simulink model "gm_CORDIC"  (R2016b)
settings: Solver=VariableStepAuto  StartTime=0.0  StopTime=20  RelTol=1e-3
undefined symbols (not defined in the file or in its folder): pht, scale, x_in, y_in, z_in
libraries: hdlsllib x24
settings Model: Creator=Arthur  LastModifiedBy=Arthur
settings OptimizationCC: BlockReduction=off  ConditionallyExecuteInputs=off
settings DebuggingCC: InheritedTsInSrcMsg=none

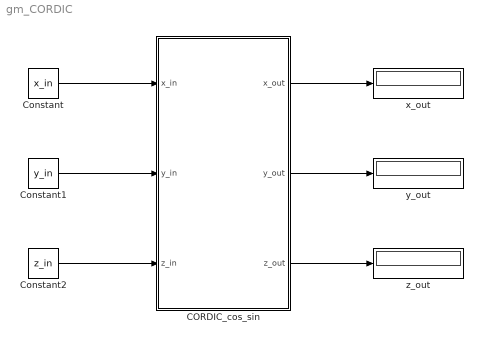
== system gm_CORDIC ==
  CORDIC_cos_sin : Subsystem
  Constant : Constant  Value=x_in  OutDataTypeStr=fixdt(1,17,14)
  Constant1 : Constant  Value=y_in  OutDataTypeStr=fixdt(1,17,14)
  Constant2 : Constant  Value=z_in  OutDataTypeStr=fixdt(1,17,14)
  x_out : Display
  y_out : Display
  z_out : Display
  wires:
  Constant/1 -> CORDIC_cos_sin/1(x_in)
  Constant1/1 -> CORDIC_cos_sin/2(y_in)
  Constant2/1 -> CORDIC_cos_sin/3(z_in)
  CORDIC_cos_sin/3(z_out) -> z_out/1
  CORDIC_cos_sin/2(y_out) -> y_out/1
  CORDIC_cos_sin/1(x_out) -> x_out/1

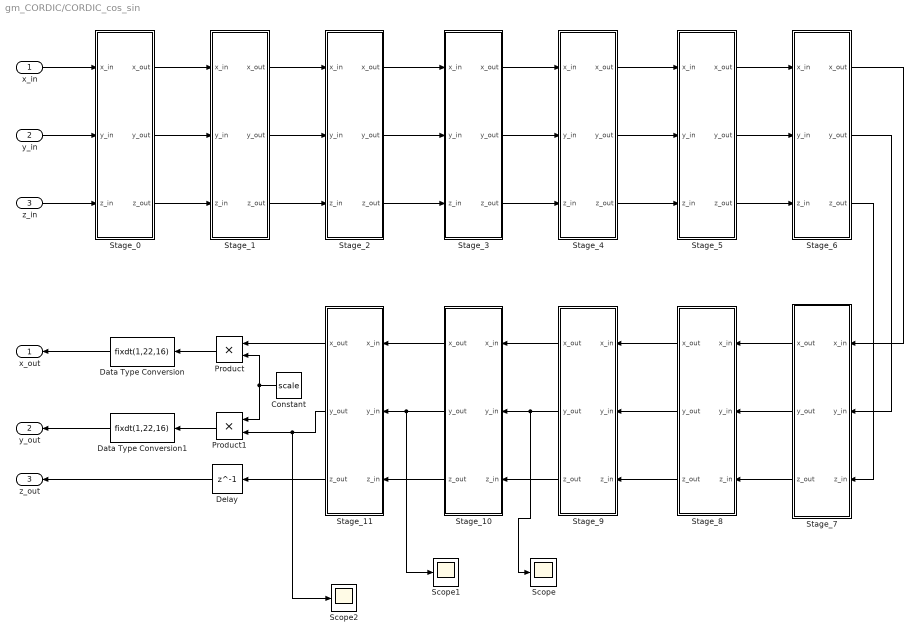
== system gm_CORDIC/CORDIC_cos_sin ==
  x_in : Inport
  y_in : Inport  Port=2
  z_in : Inport  Port=3
  Constant : Constant  Value=scale  OutDataTypeStr=fixdt(0,32,32)
  Data Type Conversion : DataTypeConversion  OutDataTypeStr=fixdt(1,22,16)
  Data Type Conversion1 : DataTypeConversion  OutDataTypeStr=fixdt(1,22,16)
  Delay : Delay  DelayLength=1
  Product : Product
  Product1 : Product
  Scope : Scope
  Scope1 : Scope
  Scope2 : Scope
  Stage_0 : Subsystem
  Stage_1 : Subsystem
  Stage_10 : Subsystem
  Stage_11 : Subsystem
  Stage_2 : Subsystem
  Stage_3 : Subsystem
  Stage_4 : Subsystem
  Stage_5 : Subsystem
  Stage_6 : Subsystem
  Stage_7 : Subsystem
  Stage_8 : Subsystem
  Stage_9 : Subsystem
  x_out : Outport
  y_out : Outport  Port=2
  z_out : Outport  Port=3
  wires:
  x_in/1 -> Stage_0/1(x_in)
  y_in/1 -> Stage_0/2(y_in)
  z_in/1 -> Stage_0/3(z_in)
  Delay/1 -> z_out/1
  Stage_5/1(x_out) -> Stage_6/1(x_in)
  Stage_4/1(x_out) -> Stage_5/1(x_in)
  Stage_3/1(x_out) -> Stage_4/1(x_in)
  Stage_2/1(x_out) -> Stage_3/1(x_in)
  Stage_1/1(x_out) -> Stage_2/1(x_in)
  Stage_1/2(y_out) -> Stage_2/2(y_in)
  Stage_2/2(y_out) -> Stage_3/2(y_in)
  Stage_3/2(y_out) -> Stage_4/2(y_in)
  Stage_4/2(y_out) -> Stage_5/2(y_in)
  Stage_5/2(y_out) -> Stage_6/2(y_in)
  Stage_5/3(z_out) -> Stage_6/3(z_in)
  Stage_4/3(z_out) -> Stage_5/3(z_in)
  Stage_3/3(z_out) -> Stage_4/3(z_in)
  Stage_2/3(z_out) -> Stage_3/3(z_in)
  Stage_1/3(z_out) -> Stage_2/3(z_in)
  Stage_0/3(z_out) -> Stage_1/3(z_in)
  Stage_0/2(y_out) -> Stage_1/2(y_in)
  Stage_0/1(x_out) -> Stage_1/1(x_in)
  Stage_6/1(x_out) -> Stage_7/1(x_in)
  Stage_6/2(y_out) -> Stage_7/2(y_in)
  Stage_6/3(z_out) -> Stage_7/3(z_in)
  Stage_10/1(x_out) -> Stage_11/1(x_in)
  Stage_10/2(y_out) -> Stage_11/2(y_in), Scope1/1
  Stage_10/3(z_out) -> Stage_11/3(z_in)
  Stage_9/3(z_out) -> Stage_10/3(z_in)
  Stage_9/2(y_out) -> Stage_10/2(y_in), Scope/1
  Stage_9/1(x_out) -> Stage_10/1(x_in)
  Stage_8/1(x_out) -> Stage_9/1(x_in)
  Stage_8/2(y_out) -> Stage_9/2(y_in)
  Stage_8/3(z_out) -> Stage_9/3(z_in)
  Stage_7/3(z_out) -> Stage_8/3(z_in)
  Stage_7/2(y_out) -> Stage_8/2(y_in)
  Stage_7/1(x_out) -> Stage_8/1(x_in)
  Stage_11/1(x_out) -> Product/1
  Stage_11/2(y_out) -> Product1/2, Scope2/1
  Stage_11/3(z_out) -> Delay/1
  Data Type Conversion1/1 -> y_out/1
  Data Type Conversion/1 -> x_out/1
  Product1/1 -> Data Type Conversion1/1
  Product/1 -> Data Type Conversion/1
  Constant/1 -> Product/2, Product1/1

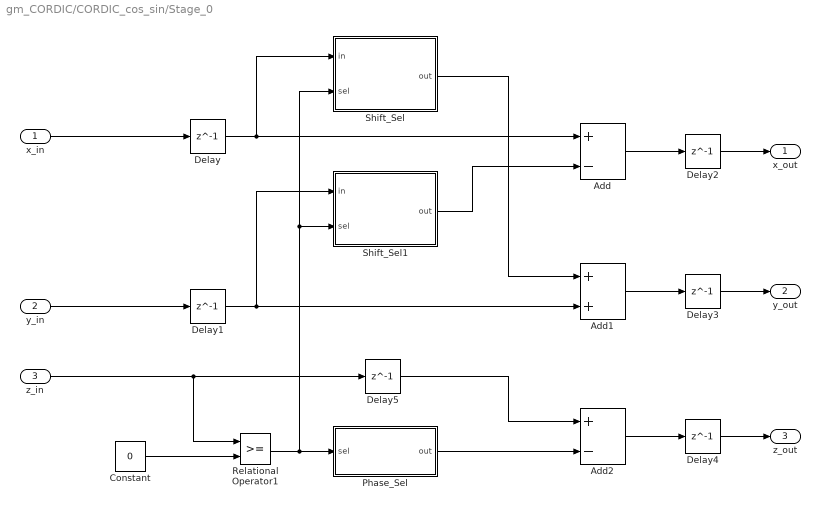
== system gm_CORDIC/CORDIC_cos_sin/Stage_0 ==
  x_in : Inport
  y_in : Inport  Port=2
  z_in : Inport  Port=3
  Add : Sum  Inputs=+-
  Add1 : Sum
  Add2 : Sum  Inputs=+-
  Constant : Constant  Value=0  OutDataTypeStr=fixdt(0,1,0)
  Delay{,1..5} (6 alike) : Delay  DelayLength=1
  Phase_Sel : Subsystem
  Relational Operator1 : RelationalOperator  OutDataTypeStr=boolean  RndMeth=Nearest
  Shift_Sel : Subsystem
  Shift_Sel1 : Subsystem
  x_out : Outport
  y_out : Outport  Port=2
  z_out : Outport  Port=3
  wires:
  Delay5/1 -> Add2/1
  Delay/1 -> Add/1, Shift_Sel/1(in)
  Phase_Sel/1(out) -> Add2/2
  Add/1 -> Delay2/1
  Add1/1 -> Delay3/1
  Delay3/1 -> y_out/1
  Add2/1 -> Delay4/1
  Delay2/1 -> x_out/1
  Delay4/1 -> z_out/1
  Shift_Sel1/1(out) -> Add/2
  z_in/1 -> Delay5/1, Relational Operator1/1
  Shift_Sel/1(out) -> Add1/1
  Delay1/1 -> Add1/2, Shift_Sel1/1(in)
  Relational Operator1/1 -> Phase_Sel/1(sel), Shift_Sel1/2(sel), Shift_Sel/2(sel)
  x_in/1 -> Delay/1
  Constant/1 -> Relational Operator1/2
  y_in/1 -> Delay1/1

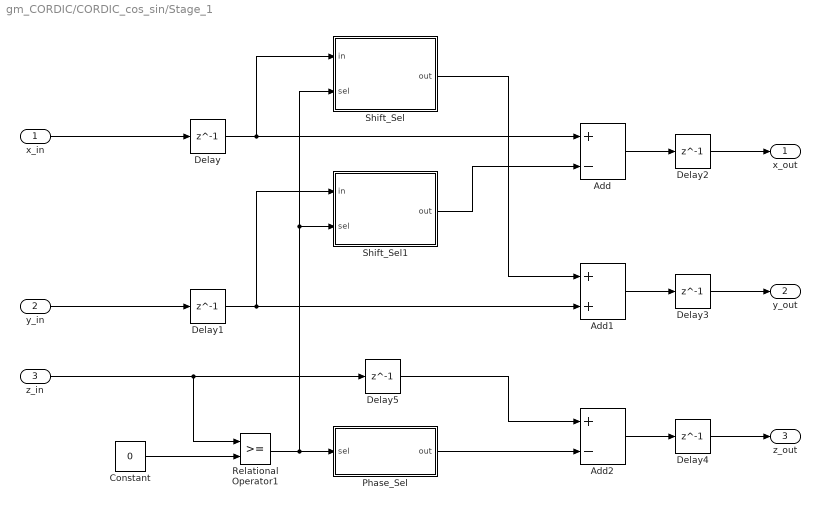
== system gm_CORDIC/CORDIC_cos_sin/Stage_1 ==
  x_in : Inport
  y_in : Inport  Port=2
  z_in : Inport  Port=3
  Add : Sum  Inputs=+-
  Add1 : Sum
  Add2 : Sum  Inputs=+-
  Constant : Constant  Value=0  OutDataTypeStr=fixdt(0,1,0)
  Delay{,1..5} (6 alike) : Delay  DelayLength=1
  Phase_Sel : Subsystem
  Relational Operator1 : RelationalOperator  OutDataTypeStr=boolean  RndMeth=Nearest
  Shift_Sel : Subsystem
  Shift_Sel1 : Subsystem
  x_out : Outport
  y_out : Outport  Port=2
  z_out : Outport  Port=3
  wires:
  Delay5/1 -> Add2/1
  Delay/1 -> Add/1, Shift_Sel/1(in)
  Phase_Sel/1(out) -> Add2/2
  Add/1 -> Delay2/1
  Add1/1 -> Delay3/1
  Delay3/1 -> y_out/1
  Add2/1 -> Delay4/1
  Delay2/1 -> x_out/1
  Delay4/1 -> z_out/1
  Shift_Sel1/1(out) -> Add/2
  z_in/1 -> Delay5/1, Relational Operator1/1
  Shift_Sel/1(out) -> Add1/1
  Delay1/1 -> Add1/2, Shift_Sel1/1(in)
  Relational Operator1/1 -> Phase_Sel/1(sel), Shift_Sel1/2(sel), Shift_Sel/2(sel)
  x_in/1 -> Delay/1
  Constant/1 -> Relational Operator1/2
  y_in/1 -> Delay1/1

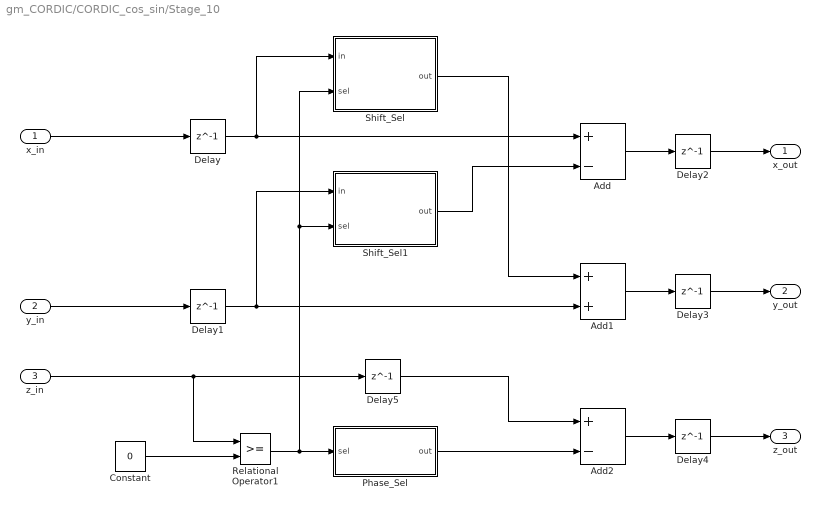
== system gm_CORDIC/CORDIC_cos_sin/Stage_10 ==
  x_in : Inport
  y_in : Inport  Port=2
  z_in : Inport  Port=3
  Add : Sum  Inputs=+-
  Add1 : Sum
  Add2 : Sum  Inputs=+-
  Constant : Constant  Value=0  OutDataTypeStr=fixdt(0,1,0)
  Delay{,1..5} (6 alike) : Delay  DelayLength=1
  Phase_Sel : Subsystem
  Relational Operator1 : RelationalOperator  OutDataTypeStr=boolean  RndMeth=Nearest
  Shift_Sel : Subsystem
  Shift_Sel1 : Subsystem
  x_out : Outport
  y_out : Outport  Port=2
  z_out : Outport  Port=3
  wires:
  Delay5/1 -> Add2/1
  Delay/1 -> Add/1, Shift_Sel/1(in)
  Phase_Sel/1(out) -> Add2/2
  Add/1 -> Delay2/1
  Add1/1 -> Delay3/1
  Delay3/1 -> y_out/1
  Add2/1 -> Delay4/1
  Delay2/1 -> x_out/1
  Delay4/1 -> z_out/1
  Shift_Sel1/1(out) -> Add/2
  z_in/1 -> Delay5/1, Relational Operator1/1
  Shift_Sel/1(out) -> Add1/1
  Delay1/1 -> Add1/2, Shift_Sel1/1(in)
  Relational Operator1/1 -> Phase_Sel/1(sel), Shift_Sel1/2(sel), Shift_Sel/2(sel)
  x_in/1 -> Delay/1
  Constant/1 -> Relational Operator1/2
  y_in/1 -> Delay1/1

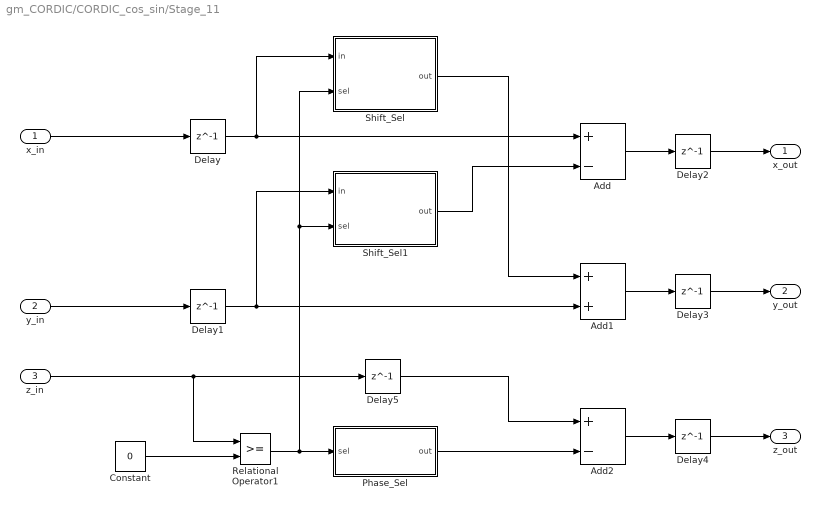
== system gm_CORDIC/CORDIC_cos_sin/Stage_11 ==
  x_in : Inport
  y_in : Inport  Port=2
  z_in : Inport  Port=3
  Add : Sum  Inputs=+-
  Add1 : Sum
  Add2 : Sum  Inputs=+-
  Constant : Constant  Value=0  OutDataTypeStr=fixdt(0,1,0)
  Delay{,1..5} (6 alike) : Delay  DelayLength=1
  Phase_Sel : Subsystem
  Relational Operator1 : RelationalOperator  OutDataTypeStr=boolean  RndMeth=Nearest
  Shift_Sel : Subsystem
  Shift_Sel1 : Subsystem
  x_out : Outport
  y_out : Outport  Port=2
  z_out : Outport  Port=3
  wires:
  Delay5/1 -> Add2/1
  Delay/1 -> Add/1, Shift_Sel/1(in)
  Phase_Sel/1(out) -> Add2/2
  Add/1 -> Delay2/1
  Add1/1 -> Delay3/1
  Delay3/1 -> y_out/1
  Add2/1 -> Delay4/1
  Delay2/1 -> x_out/1
  Delay4/1 -> z_out/1
  Shift_Sel1/1(out) -> Add/2
  z_in/1 -> Delay5/1, Relational Operator1/1
  Shift_Sel/1(out) -> Add1/1
  Delay1/1 -> Add1/2, Shift_Sel1/1(in)
  Relational Operator1/1 -> Phase_Sel/1(sel), Shift_Sel1/2(sel), Shift_Sel/2(sel)
  x_in/1 -> Delay/1
  Constant/1 -> Relational Operator1/2
  y_in/1 -> Delay1/1

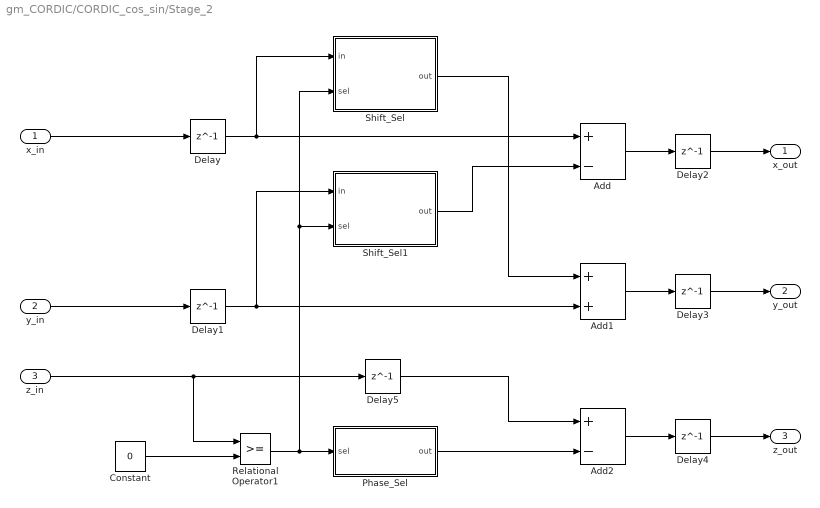
== system gm_CORDIC/CORDIC_cos_sin/Stage_2 ==
  x_in : Inport
  y_in : Inport  Port=2
  z_in : Inport  Port=3
  Add : Sum  Inputs=+-
  Add1 : Sum
  Add2 : Sum  Inputs=+-
  Constant : Constant  Value=0  OutDataTypeStr=fixdt(0,1,0)
  Delay{,1..5} (6 alike) : Delay  DelayLength=1
  Phase_Sel : Subsystem
  Relational Operator1 : RelationalOperator  OutDataTypeStr=boolean  RndMeth=Nearest
  Shift_Sel : Subsystem
  Shift_Sel1 : Subsystem
  x_out : Outport
  y_out : Outport  Port=2
  z_out : Outport  Port=3
  wires:
  Delay5/1 -> Add2/1
  Delay/1 -> Add/1, Shift_Sel/1(in)
  Phase_Sel/1(out) -> Add2/2
  Add/1 -> Delay2/1
  Add1/1 -> Delay3/1
  Delay3/1 -> y_out/1
  Add2/1 -> Delay4/1
  Delay2/1 -> x_out/1
  Delay4/1 -> z_out/1
  Shift_Sel1/1(out) -> Add/2
  z_in/1 -> Delay5/1, Relational Operator1/1
  Shift_Sel/1(out) -> Add1/1
  Delay1/1 -> Add1/2, Shift_Sel1/1(in)
  Relational Operator1/1 -> Phase_Sel/1(sel), Shift_Sel1/2(sel), Shift_Sel/2(sel)
  x_in/1 -> Delay/1
  Constant/1 -> Relational Operator1/2
  y_in/1 -> Delay1/1

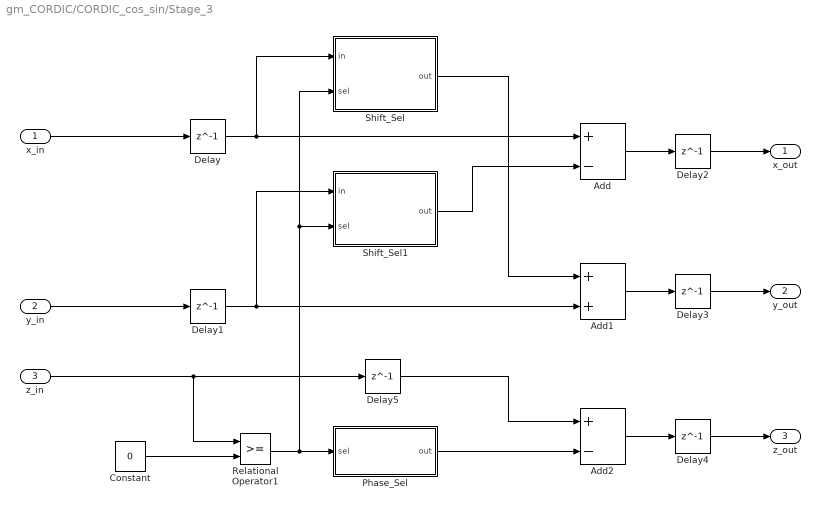
== system gm_CORDIC/CORDIC_cos_sin/Stage_3 ==
  x_in : Inport
  y_in : Inport  Port=2
  z_in : Inport  Port=3
  Add : Sum  Inputs=+-
  Add1 : Sum
  Add2 : Sum  Inputs=+-
  Constant : Constant  Value=0  OutDataTypeStr=fixdt(0,1,0)
  Delay{,1..5} (6 alike) : Delay  DelayLength=1
  Phase_Sel : Subsystem
  Relational Operator1 : RelationalOperator  OutDataTypeStr=boolean  RndMeth=Nearest
  Shift_Sel : Subsystem
  Shift_Sel1 : Subsystem
  x_out : Outport
  y_out : Outport  Port=2
  z_out : Outport  Port=3
  wires:
  Delay5/1 -> Add2/1
  Delay/1 -> Add/1, Shift_Sel/1(in)
  Phase_Sel/1(out) -> Add2/2
  Add/1 -> Delay2/1
  Add1/1 -> Delay3/1
  Delay3/1 -> y_out/1
  Add2/1 -> Delay4/1
  Delay2/1 -> x_out/1
  Delay4/1 -> z_out/1
  Shift_Sel1/1(out) -> Add/2
  z_in/1 -> Delay5/1, Relational Operator1/1
  Shift_Sel/1(out) -> Add1/1
  Delay1/1 -> Add1/2, Shift_Sel1/1(in)
  Relational Operator1/1 -> Phase_Sel/1(sel), Shift_Sel1/2(sel), Shift_Sel/2(sel)
  x_in/1 -> Delay/1
  Constant/1 -> Relational Operator1/2
  y_in/1 -> Delay1/1

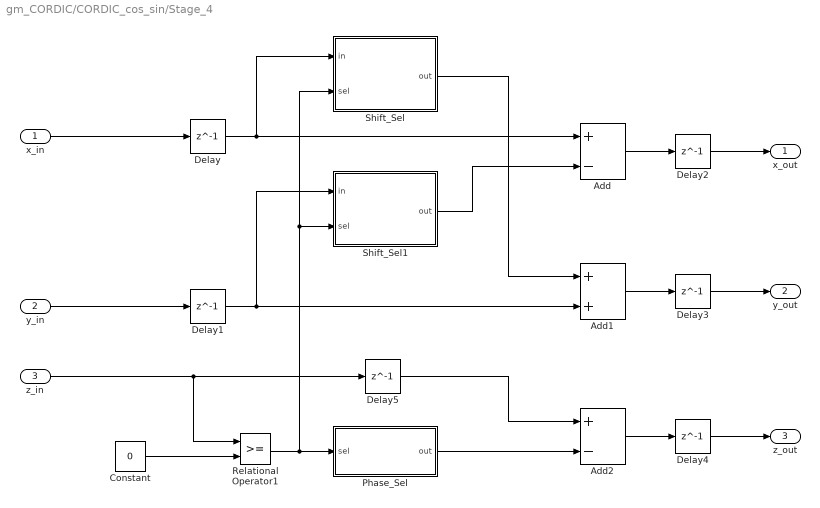
== system gm_CORDIC/CORDIC_cos_sin/Stage_4 ==
  x_in : Inport
  y_in : Inport  Port=2
  z_in : Inport  Port=3
  Add : Sum  Inputs=+-
  Add1 : Sum
  Add2 : Sum  Inputs=+-
  Constant : Constant  Value=0  OutDataTypeStr=fixdt(0,1,0)
  Delay{,1..5} (6 alike) : Delay  DelayLength=1
  Phase_Sel : Subsystem
  Relational Operator1 : RelationalOperator  OutDataTypeStr=boolean  RndMeth=Nearest
  Shift_Sel : Subsystem
  Shift_Sel1 : Subsystem
  x_out : Outport
  y_out : Outport  Port=2
  z_out : Outport  Port=3
  wires:
  Delay5/1 -> Add2/1
  Delay/1 -> Add/1, Shift_Sel/1(in)
  Phase_Sel/1(out) -> Add2/2
  Add/1 -> Delay2/1
  Add1/1 -> Delay3/1
  Delay3/1 -> y_out/1
  Add2/1 -> Delay4/1
  Delay2/1 -> x_out/1
  Delay4/1 -> z_out/1
  Shift_Sel1/1(out) -> Add/2
  z_in/1 -> Delay5/1, Relational Operator1/1
  Shift_Sel/1(out) -> Add1/1
  Delay1/1 -> Add1/2, Shift_Sel1/1(in)
  Relational Operator1/1 -> Phase_Sel/1(sel), Shift_Sel1/2(sel), Shift_Sel/2(sel)
  x_in/1 -> Delay/1
  Constant/1 -> Relational Operator1/2
  y_in/1 -> Delay1/1

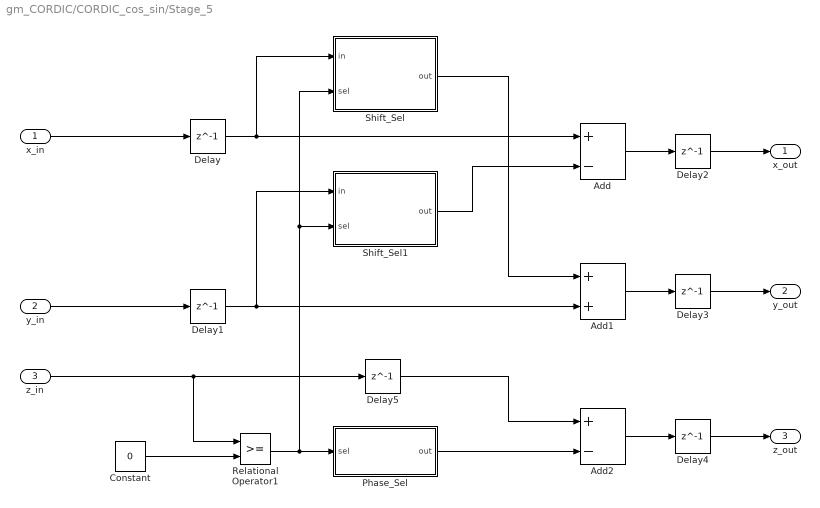
== system gm_CORDIC/CORDIC_cos_sin/Stage_5 ==
  x_in : Inport
  y_in : Inport  Port=2
  z_in : Inport  Port=3
  Add : Sum  Inputs=+-
  Add1 : Sum
  Add2 : Sum  Inputs=+-
  Constant : Constant  Value=0  OutDataTypeStr=fixdt(0,1,0)
  Delay{,1..5} (6 alike) : Delay  DelayLength=1
  Phase_Sel : Subsystem
  Relational Operator1 : RelationalOperator  OutDataTypeStr=boolean  RndMeth=Nearest
  Shift_Sel : Subsystem
  Shift_Sel1 : Subsystem
  x_out : Outport
  y_out : Outport  Port=2
  z_out : Outport  Port=3
  wires:
  Delay5/1 -> Add2/1
  Delay/1 -> Add/1, Shift_Sel/1(in)
  Phase_Sel/1(out) -> Add2/2
  Add/1 -> Delay2/1
  Add1/1 -> Delay3/1
  Delay3/1 -> y_out/1
  Add2/1 -> Delay4/1
  Delay2/1 -> x_out/1
  Delay4/1 -> z_out/1
  Shift_Sel1/1(out) -> Add/2
  z_in/1 -> Delay5/1, Relational Operator1/1
  Shift_Sel/1(out) -> Add1/1
  Delay1/1 -> Add1/2, Shift_Sel1/1(in)
  Relational Operator1/1 -> Phase_Sel/1(sel), Shift_Sel1/2(sel), Shift_Sel/2(sel)
  x_in/1 -> Delay/1
  Constant/1 -> Relational Operator1/2
  y_in/1 -> Delay1/1

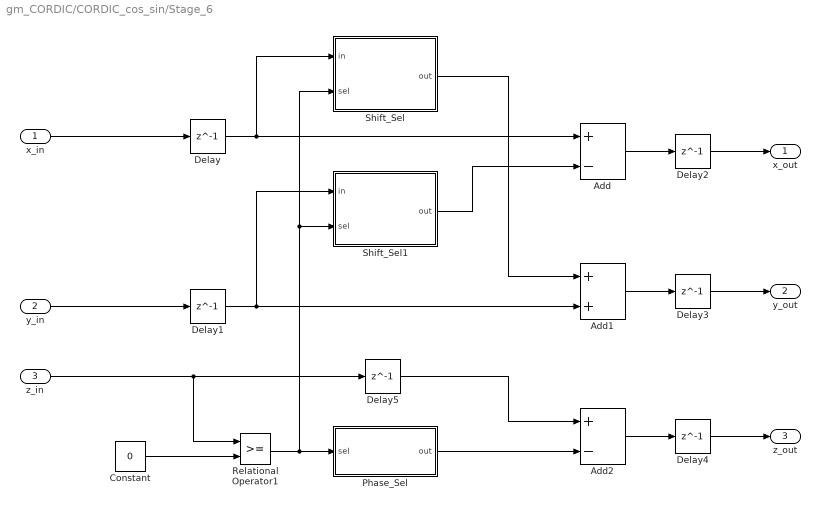
== system gm_CORDIC/CORDIC_cos_sin/Stage_6 ==
  x_in : Inport
  y_in : Inport  Port=2
  z_in : Inport  Port=3
  Add : Sum  Inputs=+-
  Add1 : Sum
  Add2 : Sum  Inputs=+-
  Constant : Constant  Value=0  OutDataTypeStr=fixdt(0,1,0)
  Delay{,1..5} (6 alike) : Delay  DelayLength=1
  Phase_Sel : Subsystem
  Relational Operator1 : RelationalOperator  OutDataTypeStr=boolean  RndMeth=Nearest
  Shift_Sel : Subsystem
  Shift_Sel1 : Subsystem
  x_out : Outport
  y_out : Outport  Port=2
  z_out : Outport  Port=3
  wires:
  Delay5/1 -> Add2/1
  Delay/1 -> Add/1, Shift_Sel/1(in)
  Phase_Sel/1(out) -> Add2/2
  Add/1 -> Delay2/1
  Add1/1 -> Delay3/1
  Delay3/1 -> y_out/1
  Add2/1 -> Delay4/1
  Delay2/1 -> x_out/1
  Delay4/1 -> z_out/1
  Shift_Sel1/1(out) -> Add/2
  z_in/1 -> Delay5/1, Relational Operator1/1
  Shift_Sel/1(out) -> Add1/1
  Delay1/1 -> Add1/2, Shift_Sel1/1(in)
  Relational Operator1/1 -> Phase_Sel/1(sel), Shift_Sel1/2(sel), Shift_Sel/2(sel)
  x_in/1 -> Delay/1
  Constant/1 -> Relational Operator1/2
  y_in/1 -> Delay1/1

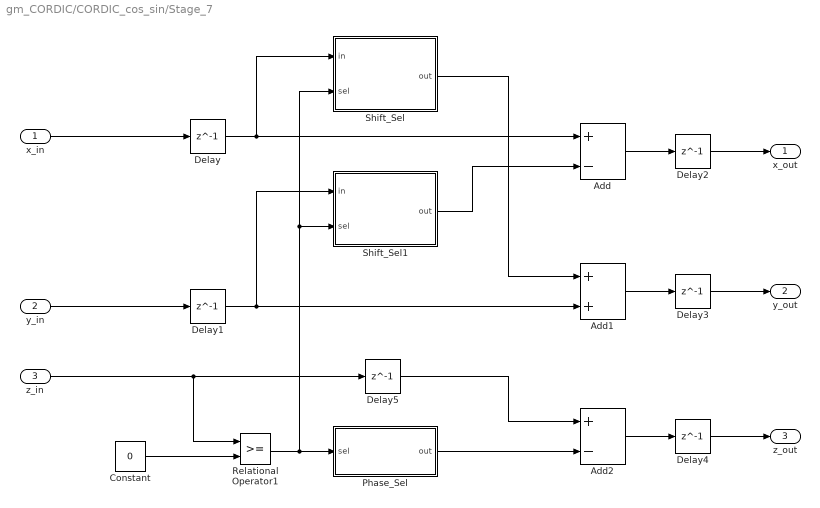
== system gm_CORDIC/CORDIC_cos_sin/Stage_7 ==
  x_in : Inport
  y_in : Inport  Port=2
  z_in : Inport  Port=3
  Add : Sum  Inputs=+-
  Add1 : Sum
  Add2 : Sum  Inputs=+-
  Constant : Constant  Value=0  OutDataTypeStr=fixdt(0,1,0)
  Delay{,1..5} (6 alike) : Delay  DelayLength=1
  Phase_Sel : Subsystem
  Relational Operator1 : RelationalOperator  OutDataTypeStr=boolean  RndMeth=Nearest
  Shift_Sel : Subsystem
  Shift_Sel1 : Subsystem
  x_out : Outport
  y_out : Outport  Port=2
  z_out : Outport  Port=3
  wires:
  Delay5/1 -> Add2/1
  Delay/1 -> Add/1, Shift_Sel/1(in)
  Phase_Sel/1(out) -> Add2/2
  Add/1 -> Delay2/1
  Add1/1 -> Delay3/1
  Delay3/1 -> y_out/1
  Add2/1 -> Delay4/1
  Delay2/1 -> x_out/1
  Delay4/1 -> z_out/1
  Shift_Sel1/1(out) -> Add/2
  z_in/1 -> Delay5/1, Relational Operator1/1
  Shift_Sel/1(out) -> Add1/1
  Delay1/1 -> Add1/2, Shift_Sel1/1(in)
  Relational Operator1/1 -> Phase_Sel/1(sel), Shift_Sel1/2(sel), Shift_Sel/2(sel)
  x_in/1 -> Delay/1
  Constant/1 -> Relational Operator1/2
  y_in/1 -> Delay1/1

== system gm_CORDIC/CORDIC_cos_sin/Stage_8 ==
  x_in : Inport
  y_in : Inport  Port=2
  z_in : Inport  Port=3
  Add : Sum  Inputs=+-
  Add1 : Sum
  Add2 : Sum  Inputs=+-
  Constant : Constant  Value=0  OutDataTypeStr=fixdt(0,1,0)
  Delay{,1..5} (6 alike) : Delay  DelayLength=1
  Phase_Sel : Subsystem
  Relational Operator1 : RelationalOperator  OutDataTypeStr=boolean  RndMeth=Nearest
  Shift_Sel : Subsystem
  Shift_Sel1 : Subsystem
  x_out : Outport
  y_out : Outport  Port=2
  z_out : Outport  Port=3
  wires:
  Delay5/1 -> Add2/1
  Delay/1 -> Add/1, Shift_Sel/1(in)
  Phase_Sel/1(out) -> Add2/2
  Add/1 -> Delay2/1
  Add1/1 -> Delay3/1
  Delay3/1 -> y_out/1
  Add2/1 -> Delay4/1
  Delay2/1 -> x_out/1
  Delay4/1 -> z_out/1
  Shift_Sel1/1(out) -> Add/2
  z_in/1 -> Delay5/1, Relational Operator1/1
  Shift_Sel/1(out) -> Add1/1
  Delay1/1 -> Add1/2, Shift_Sel1/1(in)
  Relational Operator1/1 -> Phase_Sel/1(sel), Shift_Sel1/2(sel), Shift_Sel/2(sel)
  x_in/1 -> Delay/1
  Constant/1 -> Relational Operator1/2
  y_in/1 -> Delay1/1

== system gm_CORDIC/CORDIC_cos_sin/Stage_9 ==
  x_in : Inport
  y_in : Inport  Port=2
  z_in : Inport  Port=3
  Add : Sum  Inputs=+-
  Add1 : Sum
  Add2 : Sum  Inputs=+-
  Constant : Constant  Value=0  OutDataTypeStr=fixdt(0,1,0)
  Delay{,1..5} (6 alike) : Delay  DelayLength=1
  Phase_Sel : Subsystem
  Relational Operator1 : RelationalOperator  OutDataTypeStr=boolean  RndMeth=Nearest
  Shift_Sel : Subsystem
  Shift_Sel1 : Subsystem
  x_out : Outport
  y_out : Outport  Port=2
  z_out : Outport  Port=3
  wires:
  Delay5/1 -> Add2/1
  Delay/1 -> Add/1, Shift_Sel/1(in)
  Phase_Sel/1(out) -> Add2/2
  Add/1 -> Delay2/1
  Add1/1 -> Delay3/1
  Delay3/1 -> y_out/1
  Add2/1 -> Delay4/1
  Delay2/1 -> x_out/1
  Delay4/1 -> z_out/1
  Shift_Sel1/1(out) -> Add/2
  z_in/1 -> Delay5/1, Relational Operator1/1
  Shift_Sel/1(out) -> Add1/1
  Delay1/1 -> Add1/2, Shift_Sel1/1(in)
  Relational Operator1/1 -> Phase_Sel/1(sel), Shift_Sel1/2(sel), Shift_Sel/2(sel)
  x_in/1 -> Delay/1
  Constant/1 -> Relational Operator1/2
  y_in/1 -> Delay1/1

== system gm_CORDIC/CORDIC_cos_sin/Stage_0/Phase_Sel ==
  sel : Inport
  Constant : Constant  Value=pht(1)  OutDataTypeStr=fixdt(1,16,15)
  Multiport Switch : MultiPortSwitch  DataPortOrder=Zero-based contiguous  Inputs=2
  Unary Minus : UnaryMinus
  out : Outport
  wires:
  Multiport Switch/1 -> out/1
  Unary Minus/1 -> Multiport Switch/2
  sel/1 -> Multiport Switch/1
  Constant/1 -> Multiport Switch/3, Unary Minus/1

== system gm_CORDIC/CORDIC_cos_sin/Stage_0/Shift_Sel ==
  in : Inport
  sel : Inport  Port=2
  Bit Shift : hdlsllib/HDL Operations/Bit Shift  mode=Shift Right Arithmetic  N=0
  Multiport Switch : MultiPortSwitch  DataPortOrder=Zero-based contiguous  Inputs=2
  Unary Minus : UnaryMinus
  out : Outport
  wires:
  Bit Shift/1 -> Multiport Switch/3, Unary Minus/1
  sel/1 -> Multiport Switch/1
  Multiport Switch/1 -> out/1
  in/1 -> Bit Shift/1
  Unary Minus/1 -> Multiport Switch/2

== system gm_CORDIC/CORDIC_cos_sin/Stage_0/Shift_Sel1 ==
  in : Inport
  sel : Inport  Port=2
  Bit Shift : hdlsllib/HDL Operations/Bit Shift  mode=Shift Right Arithmetic  N=0
  Multiport Switch : MultiPortSwitch  DataPortOrder=Zero-based contiguous  Inputs=2
  Unary Minus : UnaryMinus
  out : Outport
  wires:
  Bit Shift/1 -> Multiport Switch/3, Unary Minus/1
  sel/1 -> Multiport Switch/1
  Multiport Switch/1 -> out/1
  in/1 -> Bit Shift/1
  Unary Minus/1 -> Multiport Switch/2

== system gm_CORDIC/CORDIC_cos_sin/Stage_1/Phase_Sel ==
  sel : Inport
  Constant : Constant  Value=pht(2)  OutDataTypeStr=fixdt(1,16,15)
  Multiport Switch : MultiPortSwitch  DataPortOrder=Zero-based contiguous  Inputs=2
  Unary Minus : UnaryMinus
  out : Outport
  wires:
  Multiport Switch/1 -> out/1
  Unary Minus/1 -> Multiport Switch/2
  sel/1 -> Multiport Switch/1
  Constant/1 -> Multiport Switch/3, Unary Minus/1

== system gm_CORDIC/CORDIC_cos_sin/Stage_1/Shift_Sel ==
  in : Inport
  sel : Inport  Port=2
  Bit Shift : hdlsllib/HDL Operations/Bit Shift  mode=Shift Right Arithmetic  N=1
  Multiport Switch : MultiPortSwitch  DataPortOrder=Zero-based contiguous  Inputs=2
  Unary Minus : UnaryMinus
  out : Outport
  wires:
  Bit Shift/1 -> Multiport Switch/3, Unary Minus/1
  sel/1 -> Multiport Switch/1
  Multiport Switch/1 -> out/1
  in/1 -> Bit Shift/1
  Unary Minus/1 -> Multiport Switch/2

== system gm_CORDIC/CORDIC_cos_sin/Stage_1/Shift_Sel1 ==
  in : Inport
  sel : Inport  Port=2
  Bit Shift : hdlsllib/HDL Operations/Bit Shift  mode=Shift Right Arithmetic  N=1
  Multiport Switch : MultiPortSwitch  DataPortOrder=Zero-based contiguous  Inputs=2
  Unary Minus : UnaryMinus
  out : Outport
  wires:
  Bit Shift/1 -> Multiport Switch/3, Unary Minus/1
  sel/1 -> Multiport Switch/1
  Multiport Switch/1 -> out/1
  in/1 -> Bit Shift/1
  Unary Minus/1 -> Multiport Switch/2

== system gm_CORDIC/CORDIC_cos_sin/Stage_10/Phase_Sel ==
  sel : Inport
  Constant : Constant  Value=pht(11)  OutDataTypeStr=fixdt(1,16,15)
  Multiport Switch : MultiPortSwitch  DataPortOrder=Zero-based contiguous  Inputs=2
  Unary Minus : UnaryMinus
  out : Outport
  wires:
  Multiport Switch/1 -> out/1
  Unary Minus/1 -> Multiport Switch/2
  sel/1 -> Multiport Switch/1
  Constant/1 -> Multiport Switch/3, Unary Minus/1

== system gm_CORDIC/CORDIC_cos_sin/Stage_10/Shift_Sel ==
  in : Inport
  sel : Inport  Port=2
  Bit Shift : hdlsllib/HDL Operations/Bit Shift  mode=Shift Right Arithmetic  N=10
  Multiport Switch : MultiPortSwitch  DataPortOrder=Zero-based contiguous  Inputs=2
  Unary Minus : UnaryMinus
  out : Outport
  wires:
  Bit Shift/1 -> Multiport Switch/3, Unary Minus/1
  sel/1 -> Multiport Switch/1
  Multiport Switch/1 -> out/1
  in/1 -> Bit Shift/1
  Unary Minus/1 -> Multiport Switch/2

== system gm_CORDIC/CORDIC_cos_sin/Stage_10/Shift_Sel1 ==
  in : Inport
  sel : Inport  Port=2
  Bit Shift : hdlsllib/HDL Operations/Bit Shift  mode=Shift Right Arithmetic  N=10
  Multiport Switch : MultiPortSwitch  DataPortOrder=Zero-based contiguous  Inputs=2
  Unary Minus : UnaryMinus
  out : Outport
  wires:
  Bit Shift/1 -> Multiport Switch/3, Unary Minus/1
  sel/1 -> Multiport Switch/1
  Multiport Switch/1 -> out/1
  in/1 -> Bit Shift/1
  Unary Minus/1 -> Multiport Switch/2

== system gm_CORDIC/CORDIC_cos_sin/Stage_11/Phase_Sel ==
  sel : Inport
  Constant : Constant  Value=pht(12)  OutDataTypeStr=fixdt(1,16,15)
  Multiport Switch : MultiPortSwitch  DataPortOrder=Zero-based contiguous  Inputs=2
  Unary Minus : UnaryMinus
  out : Outport
  wires:
  Multiport Switch/1 -> out/1
  Unary Minus/1 -> Multiport Switch/2
  sel/1 -> Multiport Switch/1
  Constant/1 -> Multiport Switch/3, Unary Minus/1

== system gm_CORDIC/CORDIC_cos_sin/Stage_11/Shift_Sel ==
  in : Inport
  sel : Inport  Port=2
  Bit Shift : hdlsllib/HDL Operations/Bit Shift  mode=Shift Right Arithmetic  N=11
  Multiport Switch : MultiPortSwitch  DataPortOrder=Zero-based contiguous  Inputs=2
  Unary Minus : UnaryMinus
  out : Outport
  wires:
  Bit Shift/1 -> Multiport Switch/3, Unary Minus/1
  sel/1 -> Multiport Switch/1
  Multiport Switch/1 -> out/1
  in/1 -> Bit Shift/1
  Unary Minus/1 -> Multiport Switch/2

== system gm_CORDIC/CORDIC_cos_sin/Stage_11/Shift_Sel1 ==
  in : Inport
  sel : Inport  Port=2
  Bit Shift : hdlsllib/HDL Operations/Bit Shift  mode=Shift Right Arithmetic  N=11
  Multiport Switch : MultiPortSwitch  DataPortOrder=Zero-based contiguous  Inputs=2
  Unary Minus : UnaryMinus
  out : Outport
  wires:
  Bit Shift/1 -> Multiport Switch/3, Unary Minus/1
  sel/1 -> Multiport Switch/1
  Multiport Switch/1 -> out/1
  in/1 -> Bit Shift/1
  Unary Minus/1 -> Multiport Switch/2

== system gm_CORDIC/CORDIC_cos_sin/Stage_2/Phase_Sel ==
  sel : Inport
  Constant : Constant  Value=pht(3)  OutDataTypeStr=fixdt(1,16,15)
  Multiport Switch : MultiPortSwitch  DataPortOrder=Zero-based contiguous  Inputs=2
  Unary Minus : UnaryMinus
  out : Outport
  wires:
  Multiport Switch/1 -> out/1
  Unary Minus/1 -> Multiport Switch/2
  sel/1 -> Multiport Switch/1
  Constant/1 -> Multiport Switch/3, Unary Minus/1

== system gm_CORDIC/CORDIC_cos_sin/Stage_2/Shift_Sel ==
  in : Inport
  sel : Inport  Port=2
  Bit Shift : hdlsllib/HDL Operations/Bit Shift  mode=Shift Right Arithmetic  N=2
  Multiport Switch : MultiPortSwitch  DataPortOrder=Zero-based contiguous  Inputs=2
  Unary Minus : UnaryMinus
  out : Outport
  wires:
  Bit Shift/1 -> Multiport Switch/3, Unary Minus/1
  sel/1 -> Multiport Switch/1
  Multiport Switch/1 -> out/1
  in/1 -> Bit Shift/1
  Unary Minus/1 -> Multiport Switch/2

== system gm_CORDIC/CORDIC_cos_sin/Stage_2/Shift_Sel1 ==
  in : Inport
  sel : Inport  Port=2
  Bit Shift : hdlsllib/HDL Operations/Bit Shift  mode=Shift Right Arithmetic  N=2
  Multiport Switch : MultiPortSwitch  DataPortOrder=Zero-based contiguous  Inputs=2
  Unary Minus : UnaryMinus
  out : Outport
  wires:
  Bit Shift/1 -> Multiport Switch/3, Unary Minus/1
  sel/1 -> Multiport Switch/1
  Multiport Switch/1 -> out/1
  in/1 -> Bit Shift/1
  Unary Minus/1 -> Multiport Switch/2

== system gm_CORDIC/CORDIC_cos_sin/Stage_3/Phase_Sel ==
  sel : Inport
  Constant : Constant  Value=pht(4)  OutDataTypeStr=fixdt(1,16,15)
  Multiport Switch : MultiPortSwitch  DataPortOrder=Zero-based contiguous  Inputs=2
  Unary Minus : UnaryMinus
  out : Outport
  wires:
  Multiport Switch/1 -> out/1
  Unary Minus/1 -> Multiport Switch/2
  sel/1 -> Multiport Switch/1
  Constant/1 -> Multiport Switch/3, Unary Minus/1

== system gm_CORDIC/CORDIC_cos_sin/Stage_3/Shift_Sel ==
  in : Inport
  sel : Inport  Port=2
  Bit Shift : hdlsllib/HDL Operations/Bit Shift  mode=Shift Right Arithmetic  N=3
  Multiport Switch : MultiPortSwitch  DataPortOrder=Zero-based contiguous  Inputs=2
  Unary Minus : UnaryMinus
  out : Outport
  wires:
  Bit Shift/1 -> Multiport Switch/3, Unary Minus/1
  sel/1 -> Multiport Switch/1
  Multiport Switch/1 -> out/1
  in/1 -> Bit Shift/1
  Unary Minus/1 -> Multiport Switch/2

== system gm_CORDIC/CORDIC_cos_sin/Stage_3/Shift_Sel1 ==
  in : Inport
  sel : Inport  Port=2
  Bit Shift : hdlsllib/HDL Operations/Bit Shift  mode=Shift Right Arithmetic  N=3
  Multiport Switch : MultiPortSwitch  DataPortOrder=Zero-based contiguous  Inputs=2
  Unary Minus : UnaryMinus
  out : Outport
  wires:
  Bit Shift/1 -> Multiport Switch/3, Unary Minus/1
  sel/1 -> Multiport Switch/1
  Multiport Switch/1 -> out/1
  in/1 -> Bit Shift/1
  Unary Minus/1 -> Multiport Switch/2

== system gm_CORDIC/CORDIC_cos_sin/Stage_4/Phase_Sel ==
  sel : Inport
  Constant : Constant  Value=pht(5)  OutDataTypeStr=fixdt(1,16,15)
  Multiport Switch : MultiPortSwitch  DataPortOrder=Zero-based contiguous  Inputs=2
  Unary Minus : UnaryMinus
  out : Outport
  wires:
  Multiport Switch/1 -> out/1
  Unary Minus/1 -> Multiport Switch/2
  sel/1 -> Multiport Switch/1
  Constant/1 -> Multiport Switch/3, Unary Minus/1

== system gm_CORDIC/CORDIC_cos_sin/Stage_4/Shift_Sel ==
  in : Inport
  sel : Inport  Port=2
  Bit Shift : hdlsllib/HDL Operations/Bit Shift  mode=Shift Right Arithmetic  N=4
  Multiport Switch : MultiPortSwitch  DataPortOrder=Zero-based contiguous  Inputs=2
  Unary Minus : UnaryMinus
  out : Outport
  wires:
  Bit Shift/1 -> Multiport Switch/3, Unary Minus/1
  sel/1 -> Multiport Switch/1
  Multiport Switch/1 -> out/1
  in/1 -> Bit Shift/1
  Unary Minus/1 -> Multiport Switch/2

== system gm_CORDIC/CORDIC_cos_sin/Stage_4/Shift_Sel1 ==
  in : Inport
  sel : Inport  Port=2
  Bit Shift : hdlsllib/HDL Operations/Bit Shift  mode=Shift Right Arithmetic  N=4
  Multiport Switch : MultiPortSwitch  DataPortOrder=Zero-based contiguous  Inputs=2
  Unary Minus : UnaryMinus
  out : Outport
  wires:
  Bit Shift/1 -> Multiport Switch/3, Unary Minus/1
  sel/1 -> Multiport Switch/1
  Multiport Switch/1 -> out/1
  in/1 -> Bit Shift/1
  Unary Minus/1 -> Multiport Switch/2

== system gm_CORDIC/CORDIC_cos_sin/Stage_5/Phase_Sel ==
  sel : Inport
  Constant : Constant  Value=pht(6)  OutDataTypeStr=fixdt(1,16,15)
  Multiport Switch : MultiPortSwitch  DataPortOrder=Zero-based contiguous  Inputs=2
  Unary Minus : UnaryMinus
  out : Outport
  wires:
  Multiport Switch/1 -> out/1
  Unary Minus/1 -> Multiport Switch/2
  sel/1 -> Multiport Switch/1
  Constant/1 -> Multiport Switch/3, Unary Minus/1

== system gm_CORDIC/CORDIC_cos_sin/Stage_5/Shift_Sel ==
  in : Inport
  sel : Inport  Port=2
  Bit Shift : hdlsllib/HDL Operations/Bit Shift  mode=Shift Right Arithmetic  N=5
  Multiport Switch : MultiPortSwitch  DataPortOrder=Zero-based contiguous  Inputs=2
  Unary Minus : UnaryMinus
  out : Outport
  wires:
  Bit Shift/1 -> Multiport Switch/3, Unary Minus/1
  sel/1 -> Multiport Switch/1
  Multiport Switch/1 -> out/1
  in/1 -> Bit Shift/1
  Unary Minus/1 -> Multiport Switch/2

== system gm_CORDIC/CORDIC_cos_sin/Stage_5/Shift_Sel1 ==
  in : Inport
  sel : Inport  Port=2
  Bit Shift : hdlsllib/HDL Operations/Bit Shift  mode=Shift Right Arithmetic  N=5
  Multiport Switch : MultiPortSwitch  DataPortOrder=Zero-based contiguous  Inputs=2
  Unary Minus : UnaryMinus
  out : Outport
  wires:
  Bit Shift/1 -> Multiport Switch/3, Unary Minus/1
  sel/1 -> Multiport Switch/1
  Multiport Switch/1 -> out/1
  in/1 -> Bit Shift/1
  Unary Minus/1 -> Multiport Switch/2

== system gm_CORDIC/CORDIC_cos_sin/Stage_6/Phase_Sel ==
  sel : Inport
  Constant : Constant  Value=pht(7)  OutDataTypeStr=fixdt(1,16,15)
  Multiport Switch : MultiPortSwitch  DataPortOrder=Zero-based contiguous  Inputs=2
  Unary Minus : UnaryMinus
  out : Outport
  wires:
  Multiport Switch/1 -> out/1
  Unary Minus/1 -> Multiport Switch/2
  sel/1 -> Multiport Switch/1
  Constant/1 -> Multiport Switch/3, Unary Minus/1

== system gm_CORDIC/CORDIC_cos_sin/Stage_6/Shift_Sel ==
  in : Inport
  sel : Inport  Port=2
  Bit Shift : hdlsllib/HDL Operations/Bit Shift  mode=Shift Right Arithmetic  N=6
  Multiport Switch : MultiPortSwitch  DataPortOrder=Zero-based contiguous  Inputs=2
  Unary Minus : UnaryMinus
  out : Outport
  wires:
  Bit Shift/1 -> Multiport Switch/3, Unary Minus/1
  sel/1 -> Multiport Switch/1
  Multiport Switch/1 -> out/1
  in/1 -> Bit Shift/1
  Unary Minus/1 -> Multiport Switch/2

== system gm_CORDIC/CORDIC_cos_sin/Stage_6/Shift_Sel1 ==
  in : Inport
  sel : Inport  Port=2
  Bit Shift : hdlsllib/HDL Operations/Bit Shift  mode=Shift Right Arithmetic  N=6
  Multiport Switch : MultiPortSwitch  DataPortOrder=Zero-based contiguous  Inputs=2
  Unary Minus : UnaryMinus
  out : Outport
  wires:
  Bit Shift/1 -> Multiport Switch/3, Unary Minus/1
  sel/1 -> Multiport Switch/1
  Multiport Switch/1 -> out/1
  in/1 -> Bit Shift/1
  Unary Minus/1 -> Multiport Switch/2

== system gm_CORDIC/CORDIC_cos_sin/Stage_7/Phase_Sel ==
  sel : Inport
  Constant : Constant  Value=pht(8)  OutDataTypeStr=fixdt(1,16,15)
  Multiport Switch : MultiPortSwitch  DataPortOrder=Zero-based contiguous  Inputs=2
  Unary Minus : UnaryMinus
  out : Outport
  wires:
  Multiport Switch/1 -> out/1
  Unary Minus/1 -> Multiport Switch/2
  sel/1 -> Multiport Switch/1
  Constant/1 -> Multiport Switch/3, Unary Minus/1

== system gm_CORDIC/CORDIC_cos_sin/Stage_7/Shift_Sel ==
  in : Inport
  sel : Inport  Port=2
  Bit Shift : hdlsllib/HDL Operations/Bit Shift  mode=Shift Right Arithmetic  N=7
  Multiport Switch : MultiPortSwitch  DataPortOrder=Zero-based contiguous  Inputs=2
  Unary Minus : UnaryMinus
  out : Outport
  wires:
  Bit Shift/1 -> Multiport Switch/3, Unary Minus/1
  sel/1 -> Multiport Switch/1
  Multiport Switch/1 -> out/1
  in/1 -> Bit Shift/1
  Unary Minus/1 -> Multiport Switch/2

== system gm_CORDIC/CORDIC_cos_sin/Stage_7/Shift_Sel1 ==
  in : Inport
  sel : Inport  Port=2
  Bit Shift : hdlsllib/HDL Operations/Bit Shift  mode=Shift Right Arithmetic  N=7
  Multiport Switch : MultiPortSwitch  DataPortOrder=Zero-based contiguous  Inputs=2
  Unary Minus : UnaryMinus
  out : Outport
  wires:
  Bit Shift/1 -> Multiport Switch/3, Unary Minus/1
  sel/1 -> Multiport Switch/1
  Multiport Switch/1 -> out/1
  in/1 -> Bit Shift/1
  Unary Minus/1 -> Multiport Switch/2

== system gm_CORDIC/CORDIC_cos_sin/Stage_8/Phase_Sel ==
  sel : Inport
  Constant : Constant  Value=pht(9)  OutDataTypeStr=fixdt(1,16,15)
  Multiport Switch : MultiPortSwitch  DataPortOrder=Zero-based contiguous  Inputs=2
  Unary Minus : UnaryMinus
  out : Outport
  wires:
  Multiport Switch/1 -> out/1
  Unary Minus/1 -> Multiport Switch/2
  sel/1 -> Multiport Switch/1
  Constant/1 -> Multiport Switch/3, Unary Minus/1

== system gm_CORDIC/CORDIC_cos_sin/Stage_8/Shift_Sel ==
  in : Inport
  sel : Inport  Port=2
  Bit Shift : hdlsllib/HDL Operations/Bit Shift  mode=Shift Right Arithmetic  N=8
  Multiport Switch : MultiPortSwitch  DataPortOrder=Zero-based contiguous  Inputs=2
  Unary Minus : UnaryMinus
  out : Outport
  wires:
  Bit Shift/1 -> Multiport Switch/3, Unary Minus/1
  sel/1 -> Multiport Switch/1
  Multiport Switch/1 -> out/1
  in/1 -> Bit Shift/1
  Unary Minus/1 -> Multiport Switch/2

== system gm_CORDIC/CORDIC_cos_sin/Stage_8/Shift_Sel1 ==
  in : Inport
  sel : Inport  Port=2
  Bit Shift : hdlsllib/HDL Operations/Bit Shift  mode=Shift Right Arithmetic  N=8
  Multiport Switch : MultiPortSwitch  DataPortOrder=Zero-based contiguous  Inputs=2
  Unary Minus : UnaryMinus
  out : Outport
  wires:
  Bit Shift/1 -> Multiport Switch/3, Unary Minus/1
  sel/1 -> Multiport Switch/1
  Multiport Switch/1 -> out/1
  in/1 -> Bit Shift/1
  Unary Minus/1 -> Multiport Switch/2

== system gm_CORDIC/CORDIC_cos_sin/Stage_9/Phase_Sel ==
  sel : Inport
  Constant : Constant  Value=pht(10)  OutDataTypeStr=fixdt(1,16,15)
  Multiport Switch : MultiPortSwitch  DataPortOrder=Zero-based contiguous  Inputs=2
  Unary Minus : UnaryMinus
  out : Outport
  wires:
  Multiport Switch/1 -> out/1
  Unary Minus/1 -> Multiport Switch/2
  sel/1 -> Multiport Switch/1
  Constant/1 -> Multiport Switch/3, Unary Minus/1

== system gm_CORDIC/CORDIC_cos_sin/Stage_9/Shift_Sel ==
  in : Inport
  sel : Inport  Port=2
  Bit Shift : hdlsllib/HDL Operations/Bit Shift  mode=Shift Right Arithmetic  N=9
  Multiport Switch : MultiPortSwitch  DataPortOrder=Zero-based contiguous  Inputs=2
  Unary Minus : UnaryMinus
  out : Outport
  wires:
  Bit Shift/1 -> Multiport Switch/3, Unary Minus/1
  sel/1 -> Multiport Switch/1
  Multiport Switch/1 -> out/1
  in/1 -> Bit Shift/1
  Unary Minus/1 -> Multiport Switch/2

== system gm_CORDIC/CORDIC_cos_sin/Stage_9/Shift_Sel1 ==
  in : Inport
  sel : Inport  Port=2
  Bit Shift : hdlsllib/HDL Operations/Bit Shift  mode=Shift Right Arithmetic  N=9
  Multiport Switch : MultiPortSwitch  DataPortOrder=Zero-based contiguous  Inputs=2
  Unary Minus : UnaryMinus
  out : Outport
  wires:
  Bit Shift/1 -> Multiport Switch/3, Unary Minus/1
  sel/1 -> Multiport Switch/1
  Multiport Switch/1 -> out/1
  in/1 -> Bit Shift/1
  Unary Minus/1 -> Multiport Switch/2
